simulink model "TwoTanks_Interact_noControl"  (R2023b)
settings: Solver=ode4  StartTime=0.0  StopTime=1/10  FixedStep=1/10  RelTol=1e-3  EnableMultiTasking=on
InitFcn:
  | init_twotanks_interact
values from neighbouring files (symbols this model uses):
  u0 = 0    [TwoTank_Simulate_NoSimulink.m]    (also in init_twotanks_interact.m = Parameters.model.control_0)
settings Model: Creator=Windows  LastModifiedBy=HP
settings SolverCC: AlgebraicLoopSolver=TrustRegion
settings DataIOCC: ReturnWorkspaceOutputs=off
settings OptimizationCC: DefaultParameterBehavior=Inlined  BufferReuse=off
settings DebuggingCC: UnconnectedInputMsg=warning  UnconnectedOutputMsg=warning  UnconnectedLineMsg=warning  InitInArrayFormatMsg=none  ArithmeticOperatorsInVariantConditions=warning
settings ModelReferenceCC: EnableRefExpFcnMdlSchedulingChecks=on
settings SFSimCC: CustomCodeUndefinedFunction=UseInterfaceOnly
settings RTWCC: DLArmComputeVersion=19.05

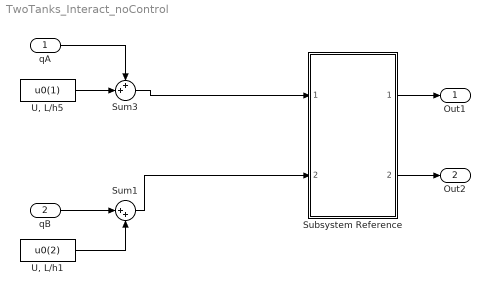
== system TwoTanks_Interact_noControl ==
  qA : Inport
  qB : Inport  Port=2
  Subsystem Reference : Subsystem  ReferencedSubsystem=TwoTanks_Sub
  Sum1 : Sum  Inputs=|++
  Sum3 : Sum  Inputs=++|
  "U, L/h1" : Constant  Value=u0(2)
  "U, L/h5" : Constant  Value=u0(1)
  Out1 : Outport  VectorParamsAs1DForOutWhenUnconnected=off
  Out2 : Outport  Port=2  VectorParamsAs1DForOutWhenUnconnected=off
  wires:
  Subsystem Reference/2 -> Out2/1
  Subsystem Reference/1 -> Out1/1
  Sum3/1 -> Subsystem Reference/1
  Sum1/1 -> Subsystem Reference/2
  "U, L/h1"/1 -> Sum1/2
  qB/1 -> Sum1/1
  qA/1 -> Sum3/1
  "U, L/h5"/1 -> Sum3/2
